simulink model "model_compatible"  (Simulink 7.5)
settings: Solver=ode45  StartTime=0.0  StopTime=10.0  RelTol=1e-3
libraries: powerlib x51
settings Model: Creator=lej  LastModifiedBy=epezhman  CovModelRefEnable=off
settings DataIOCC: SaveFormat=StructureWithTime
settings OptimizationCC: ExpressionDepthLimit=128
settings DebuggingCC: UnderspecifiedInitializationDetection=Simplified  MergeDetectMultiDrivingBlocksExec=error  SolverPrmCheckMsg=none  FcnCallInpInsideContextMsg=Enable All  StateNameClashWarn=none
settings HardwareCC: ProdIntDivRoundTo=Zero  ProdEndianess=LittleEndian  ProdHWDeviceType=Specified
settings CodeAppCC: CustomSymbolStrType=$N$R$M_T
settings GRTTargetCC: TargetFunctionLibrary=C89/C90 (ANSI)  GeneratePreprocessorConditionals=Use local settings

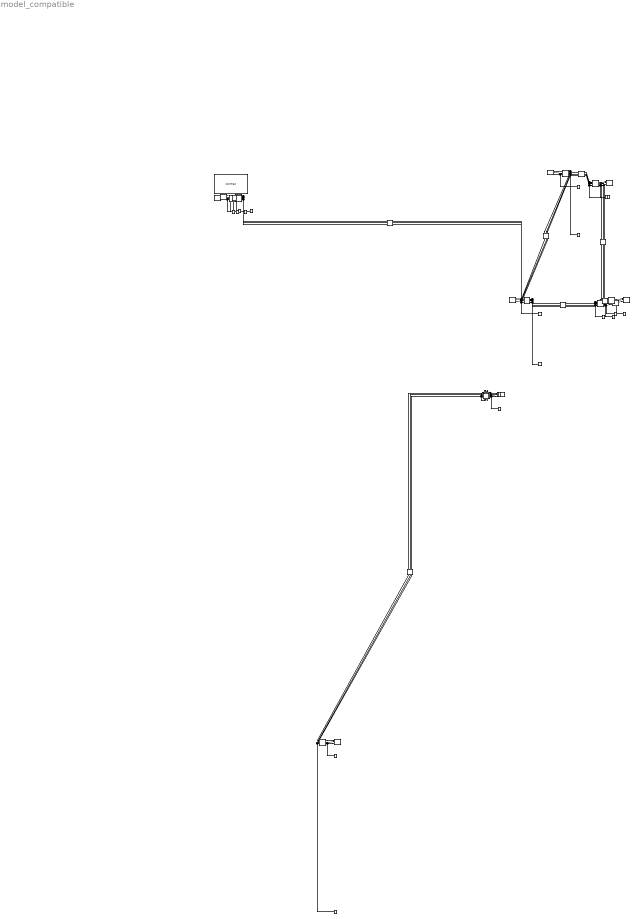
== system model_compatible ==
  note: 220000 Volts Power Line
  G_179496206_ : powerlib/Electrical Sources/Three-Phase Source  InternalConnection=Yg  VoltagePhases=off  Voltage=220000  PhaseAngle=0  Voltage_phases=[ 1 1 1]*380000  PhaseAngles_phases=[ 0 0 0]  Frequency=50  NonIdealSource=on  SpecifyImpedance=off  Resistance=0.8929  Inductance=16.58e-3  ShortCircuitLevel=100e6  BaseVoltage=220000  XRratio=7  BusType=swing  Pref=90000000  Qref=0  Prefabc=[3333.33 3333.33 3333.33]  Qrefabc=[0 0 0]  Qmin=-inf  Qmax=inf
  G_179509355_ : powerlib/Electrical Sources/Three-Phase Source  InternalConnection=Yg  VoltagePhases=off  Voltage=220000  PhaseAngle=0  Voltage_phases=[ 1 1 1]*380000  PhaseAngles_phases=[ 0 0 0]  Frequency=50  NonIdealSource=on  SpecifyImpedance=off  Resistance=0.8929  Inductance=16.58e-3  ShortCircuitLevel=100e6  BaseVoltage=220000  XRratio=7  BusType=swing  Pref=133000000  Qref=0  Prefabc=[3333.33 3333.33 3333.33]  Qrefabc=[0 0 0]  Qmin=-inf  Qmax=inf
  L_{179488572,179490334,179490336,179496196..179496198,179496204,179509359,179509364} (9 alike) : powerlib/Elements/Three-Phase Series RLC Load  LConnTagsString=A|B|C  Configuration=Y (grounded)  NominalVoltage=220000  Vabc=[1e3 1e3 1e3]  Vabcp=[1e3 1e3 1e3]  NominalFrequency=50  UnbalancedPower=off  ActivePower=100000  InductivePower=100  CapacitivePower=100  Pabc=[10e3 9e3 11e3]  QLabc=[100 90 110]  QCabc=[100 90 110]  Pabcp=[10e3 9e3 11e3]  QLabcp=[100 90 110]  QCabcp=[100 90 110]  Measurements=None  LoadType=constant PQ
  T_179488572_400000;220000_Phokoje_Substation : powerlib/Elements/Three-Phase Transformer (Two Windings)  Winding1Connection=Yg  Winding2Connection=Yg  CoreType=Three single-phase transformers  SetSaturation=off  Hysteresis=off  DataFile='hysteresis'  SetInitialFlux=off  Measurements=None  UNITS=pu  NominalPower=[ 250e6 , 50 ]  Winding1=[220000,0.002,0.08]  Winding2=[220000,0.002,0.08]  Rm=2000  Lm=50  L0=0.5  Saturation=[ 0,0 ; 0.0024,1.2 ; 1.0,1.52 ]  InitialFluxes=[ 0.8 , -0.8 , 0.7 ]  MoreParameters=off  BreakLoop=off  DataType=off  TransfoNumber=1
  T_179490334_220000_Tati_Substation : powerlib/Elements/Three-Phase Transformer (Two Windings)  Winding1Connection=Yg  Winding2Connection=Yg  CoreType=Three single-phase transformers  SetSaturation=off  Hysteresis=off  DataFile='hysteresis'  SetInitialFlux=off  Measurements=None  UNITS=pu  NominalPower=[ 250e6 , 50 ]  Winding1=[220000,0.002,0.08]  Winding2=[220000,0.002,0.08]  Rm=2000  Lm=50  L0=0.5  Saturation=[ 0,0 ; 0.0024,1.2 ; 1.0,1.52 ]  InitialFluxes=[ 0.8 , -0.8 , 0.7 ]  MoreParameters=off  BreakLoop=off  DataType=off  TransfoNumber=1
  T_179490336_220000_Francistown_Substation : powerlib/Elements/Three-Phase Transformer (Two Windings)  Winding1Connection=Yg  Winding2Connection=Yg  CoreType=Three single-phase transformers  SetSaturation=off  Hysteresis=off  DataFile='hysteresis'  SetInitialFlux=off  Measurements=None  UNITS=pu  NominalPower=[ 250e6 , 50 ]  Winding1=[220000,0.002,0.08]  Winding2=[220000,0.002,0.08]  Rm=2000  Lm=50  L0=0.5  Saturation=[ 0,0 ; 0.0024,1.2 ; 1.0,1.52 ]  InitialFluxes=[ 0.8 , -0.8 , 0.7 ]  MoreParameters=off  BreakLoop=off  DataType=off  TransfoNumber=1
  T_179496196_220000_Selebi_Pikwe_Substation : powerlib/Elements/Three-Phase Transformer (Two Windings)  Winding1Connection=Yg  Winding2Connection=Yg  CoreType=Three single-phase transformers  SetSaturation=off  Hysteresis=off  DataFile='hysteresis'  SetInitialFlux=off  Measurements=None  UNITS=pu  NominalPower=[ 250e6 , 50 ]  Winding1=[220000,0.002,0.08]  Winding2=[220000,0.002,0.08]  Rm=2000  Lm=50  L0=0.5  Saturation=[ 0,0 ; 0.0024,1.2 ; 1.0,1.52 ]  InitialFluxes=[ 0.8 , -0.8 , 0.7 ]  MoreParameters=off  BreakLoop=off  DataType=off  TransfoNumber=1
  T_179496197_220000_Orapa_Substation : powerlib/Elements/Three-Phase Transformer (Two Windings)  Winding1Connection=Yg  Winding2Connection=Yg  CoreType=Three single-phase transformers  SetSaturation=off  Hysteresis=off  DataFile='hysteresis'  SetInitialFlux=off  Measurements=None  UNITS=pu  NominalPower=[ 250e6 , 50 ]  Winding1=[220000,0.002,0.08]  Winding2=[220000,0.002,0.08]  Rm=2000  Lm=50  L0=0.5  Saturation=[ 0,0 ; 0.0024,1.2 ; 1.0,1.52 ]  InitialFluxes=[ 0.8 , -0.8 , 0.7 ]  MoreParameters=off  BreakLoop=off  DataType=off  TransfoNumber=1
  T_179496198_220000_Serule_Substation : powerlib/Elements/Three-Phase Transformer (Two Windings)  Winding1Connection=Yg  Winding2Connection=Yg  CoreType=Three single-phase transformers  SetSaturation=off  Hysteresis=off  DataFile='hysteresis'  SetInitialFlux=off  Measurements=None  UNITS=pu  NominalPower=[ 250e6 , 50 ]  Winding1=[220000,0.002,0.08]  Winding2=[220000,0.002,0.08]  Rm=2000  Lm=50  L0=0.5  Saturation=[ 0,0 ; 0.0024,1.2 ; 1.0,1.52 ]  InitialFluxes=[ 0.8 , -0.8 , 0.7 ]  MoreParameters=off  BreakLoop=off  DataType=off  TransfoNumber=1
  T_179496204_220000_Orapa_Substation : powerlib/Elements/Three-Phase Transformer (Two Windings)  Winding1Connection=Yg  Winding2Connection=Yg  CoreType=Three single-phase transformers  SetSaturation=off  Hysteresis=off  DataFile='hysteresis'  SetInitialFlux=off  Measurements=None  UNITS=pu  NominalPower=[ 250e6 , 50 ]  Winding1=[220000,0.002,0.08]  Winding2=[220000,0.002,0.08]  Rm=2000  Lm=50  L0=0.5  Saturation=[ 0,0 ; 0.0024,1.2 ; 1.0,1.52 ]  InitialFluxes=[ 0.8 , -0.8 , 0.7 ]  MoreParameters=off  BreakLoop=off  DataType=off  TransfoNumber=1
  T_179509359__ : powerlib/Elements/Three-Phase Transformer (Two Windings)  Winding1Connection=Yg  Winding2Connection=Yg  CoreType=Three single-phase transformers  SetSaturation=off  Hysteresis=off  DataFile='hysteresis'  SetInitialFlux=off  Measurements=None  UNITS=pu  NominalPower=[ 250e6 , 50 ]  Winding1=[220000,0.002,0.08]  Winding2=[220000,0.002,0.08]  Rm=2000  Lm=50  L0=0.5  Saturation=[ 0,0 ; 0.0024,1.2 ; 1.0,1.52 ]  InitialFluxes=[ 0.8 , -0.8 , 0.7 ]  MoreParameters=off  BreakLoop=off  DataType=off  TransfoNumber=1
  T_179509364_220000_Gaborone_Substation : powerlib/Elements/Three-Phase Transformer (Two Windings)  Winding1Connection=Yg  Winding2Connection=Yg  CoreType=Three single-phase transformers  SetSaturation=off  Hysteresis=off  DataFile='hysteresis'  SetInitialFlux=off  Measurements=None  UNITS=pu  NominalPower=[ 250e6 , 50 ]  Winding1=[220000,0.002,0.08]  Winding2=[220000,0.002,0.08]  Rm=2000  Lm=50  L0=0.5  Saturation=[ 0,0 ; 0.0024,1.2 ; 1.0,1.52 ]  InitialFluxes=[ 0.8 , -0.8 , 0.7 ]  MoreParameters=off  BreakLoop=off  DataType=off  TransfoNumber=1
  _CN_179488572_220000_CN_179490334_220000 : powerlib/Elements/Distributed Parameters Line  Phases=3  Frequency=50  Resistance=[0.01273 0.3864]  Inductance="[0.9337e-3  4.1264e-3]"  Capacitance=[12.74e-9 7.751e-9]  Length=84.299  x1=[8.73114913702011e-11 380000 380000;314.159265358979 314.159265358979 314.159265358979;-0.177670123217348 0.415246442777429 -1.15554988401747]  x2=[1.26090477118469e-09 381852.398472139 381852.398472139;314.159265358979 314.159265358979 314.159265358979;-1.41941675517191 0.415007521738739 -1.15578880505616]  x3=[1.07663708898761e-11 1405.24743813465 1405.24743813466;314.159265358979 314.159265358979 314.159265358979;-2.70558821102223 0.316110507002444 -1.25468581979246]  x4=[8.62234243168895e-12 1405.96374414071 1405.9637441407;314.159265358979 314.159265358979 314.159265358979;0.245769282942371 0.405640215255436 -1.16515611153945]  x5=0.000565541566995742  V1=ones(3,3)  V2=ones(3,3)  I1=ones(3,3)  I2=ones(3,3)  nHarmo=1  Measurements=None
  _CN_179490336_220000_CN_179490334_220000 : powerlib/Elements/Distributed Parameters Line  Phases=3  Frequency=50  Resistance=[0.01273 0.3864]  Inductance="[0.9337e-3  4.1264e-3]"  Capacitance=[12.74e-9 7.751e-9]  Length=27.304  x1=[8.73114913702011e-11 380000 380000;314.159265358979 314.159265358979 314.159265358979;-0.177670123217348 0.415246442777429 -1.15554988401747]  x2=[1.26090477118469e-09 381852.398472139 381852.398472139;314.159265358979 314.159265358979 314.159265358979;-1.41941675517191 0.415007521738739 -1.15578880505616]  x3=[1.07663708898761e-11 1405.24743813465 1405.24743813466;314.159265358979 314.159265358979 314.159265358979;-2.70558821102223 0.316110507002444 -1.25468581979246]  x4=[8.62234243168895e-12 1405.96374414071 1405.9637441407;314.159265358979 314.159265358979 314.159265358979;0.245769282942371 0.405640215255436 -1.16515611153945]  x5=0.000565541566995742  V1=ones(3,3)  V2=ones(3,3)  I1=ones(3,3)  I2=ones(3,3)  nHarmo=1  Measurements=None
  _CN_179490336_220000_CN_179496198_220000 : powerlib/Elements/Distributed Parameters Line  Phases=3  Frequency=50  Resistance=[0.01273 0.3864]  Inductance="[0.9337e-3  4.1264e-3]"  Capacitance=[12.74e-9 7.751e-9]  Length=92.6463  x1=[8.73114913702011e-11 380000 380000;314.159265358979 314.159265358979 314.159265358979;-0.177670123217348 0.415246442777429 -1.15554988401747]  x2=[1.26090477118469e-09 381852.398472139 381852.398472139;314.159265358979 314.159265358979 314.159265358979;-1.41941675517191 0.415007521738739 -1.15578880505616]  x3=[1.07663708898761e-11 1405.24743813465 1405.24743813466;314.159265358979 314.159265358979 314.159265358979;-2.70558821102223 0.316110507002444 -1.25468581979246]  x4=[8.62234243168895e-12 1405.96374414071 1405.9637441407;314.159265358979 314.159265358979 314.159265358979;0.245769282942371 0.405640215255436 -1.16515611153945]  x5=0.000565541566995742  V1=ones(3,3)  V2=ones(3,3)  I1=ones(3,3)  I2=ones(3,3)  nHarmo=1  Measurements=None
  _CN_179496196_220000_CN_179488572_220000 : powerlib/Elements/Distributed Parameters Line  Phases=3  Frequency=50  Resistance=[0.01273 0.3864]  Inductance="[0.9337e-3  4.1264e-3]"  Capacitance=[12.74e-9 7.751e-9]  Length=7.9024  x1=[8.73114913702011e-11 380000 380000;314.159265358979 314.159265358979 314.159265358979;-0.177670123217348 0.415246442777429 -1.15554988401747]  x2=[1.26090477118469e-09 381852.398472139 381852.398472139;314.159265358979 314.159265358979 314.159265358979;-1.41941675517191 0.415007521738739 -1.15578880505616]  x3=[1.07663708898761e-11 1405.24743813465 1405.24743813466;314.159265358979 314.159265358979 314.159265358979;-2.70558821102223 0.316110507002444 -1.25468581979246]  x4=[8.62234243168895e-12 1405.96374414071 1405.9637441407;314.159265358979 314.159265358979 314.159265358979;0.245769282942371 0.405640215255436 -1.16515611153945]  x5=0.000565541566995742  V1=ones(3,3)  V2=ones(3,3)  I1=ones(3,3)  I2=ones(3,3)  nHarmo=1  Measurements=None
  _CN_179496197_220000_CN_179496204_220000 : powerlib/Elements/Distributed Parameters Line  Phases=3  Frequency=50  Resistance=[0.01273 0.3864]  Inductance="[0.9337e-3  4.1264e-3]"  Capacitance=[12.74e-9 7.751e-9]  Length=4.007  x1=[8.73114913702011e-11 380000 380000;314.159265358979 314.159265358979 314.159265358979;-0.177670123217348 0.415246442777429 -1.15554988401747]  x2=[1.26090477118469e-09 381852.398472139 381852.398472139;314.159265358979 314.159265358979 314.159265358979;-1.41941675517191 0.415007521738739 -1.15578880505616]  x3=[1.07663708898761e-11 1405.24743813465 1405.24743813466;314.159265358979 314.159265358979 314.159265358979;-2.70558821102223 0.316110507002444 -1.25468581979246]  x4=[8.62234243168895e-12 1405.96374414071 1405.9637441407;314.159265358979 314.159265358979 314.159265358979;0.245769282942371 0.405640215255436 -1.16515611153945]  x5=0.000565541566995742  V1=ones(3,3)  V2=ones(3,3)  I1=ones(3,3)  I2=ones(3,3)  nHarmo=1  Measurements=None
  _CN_179496198_220000_CN_179488572_220000 : powerlib/Elements/Distributed Parameters Line  Phases=3  Frequency=50  Resistance=[0.01273 0.3864]  Inductance="[0.9337e-3  4.1264e-3]"  Capacitance=[12.74e-9 7.751e-9]  Length=51.2709  x1=[8.73114913702011e-11 380000 380000;314.159265358979 314.159265358979 314.159265358979;-0.177670123217348 0.415246442777429 -1.15554988401747]  x2=[1.26090477118469e-09 381852.398472139 381852.398472139;314.159265358979 314.159265358979 314.159265358979;-1.41941675517191 0.415007521738739 -1.15578880505616]  x3=[1.07663708898761e-11 1405.24743813465 1405.24743813466;314.159265358979 314.159265358979 314.159265358979;-2.70558821102223 0.316110507002444 -1.25468581979246]  x4=[8.62234243168895e-12 1405.96374414071 1405.9637441407;314.159265358979 314.159265358979 314.159265358979;0.245769282942371 0.405640215255436 -1.16515611153945]  x5=0.000565541566995742  V1=ones(3,3)  V2=ones(3,3)  I1=ones(3,3)  I2=ones(3,3)  nHarmo=1  Measurements=None
  _CN_179496198_220000_CN_179496204_220000 : powerlib/Elements/Distributed Parameters Line  Phases=3  Frequency=50  Resistance=[0.01273 0.3864]  Inductance="[0.9337e-3  4.1264e-3]"  Capacitance=[12.74e-9 7.751e-9]  Length=33.2853  x1=[8.73114913702011e-11 380000 380000;314.159265358979 314.159265358979 314.159265358979;-0.177670123217348 0.415246442777429 -1.15554988401747]  x2=[1.26090477118469e-09 381852.398472139 381852.398472139;314.159265358979 314.159265358979 314.159265358979;-1.41941675517191 0.415007521738739 -1.15578880505616]  x3=[1.07663708898761e-11 1405.24743813465 1405.24743813466;314.159265358979 314.159265358979 314.159265358979;-2.70558821102223 0.316110507002444 -1.25468581979246]  x4=[8.62234243168895e-12 1405.96374414071 1405.9637441407;314.159265358979 314.159265358979 314.159265358979;0.245769282942371 0.405640215255436 -1.16515611153945]  x5=0.000565541566995742  V1=ones(3,3)  V2=ones(3,3)  I1=ones(3,3)  I2=ones(3,3)  nHarmo=1  Measurements=None
  _CN_179496204_220000_CN_179496206_220000 : powerlib/Elements/Distributed Parameters Line  Phases=3  Frequency=50  Resistance=[0.01273 0.3864]  Inductance="[0.9337e-3  4.1264e-3]"  Capacitance=[12.74e-9 7.751e-9]  Length=0.29284  x1=[8.73114913702011e-11 380000 380000;314.159265358979 314.159265358979 314.159265358979;-0.177670123217348 0.415246442777429 -1.15554988401747]  x2=[1.26090477118469e-09 381852.398472139 381852.398472139;314.159265358979 314.159265358979 314.159265358979;-1.41941675517191 0.415007521738739 -1.15578880505616]  x3=[1.07663708898761e-11 1405.24743813465 1405.24743813466;314.159265358979 314.159265358979 314.159265358979;-2.70558821102223 0.316110507002444 -1.25468581979246]  x4=[8.62234243168895e-12 1405.96374414071 1405.9637441407;314.159265358979 314.159265358979 314.159265358979;0.245769282942371 0.405640215255436 -1.16515611153945]  x5=0.000565541566995742  V1=ones(3,3)  V2=ones(3,3)  I1=ones(3,3)  I2=ones(3,3)  nHarmo=1  Measurements=None
  _CN_179509359_220000_CN_179509355_220000 : powerlib/Elements/Distributed Parameters Line  Phases=3  Frequency=50  Resistance=[0.01273 0.3864]  Inductance="[0.9337e-3  4.1264e-3]"  Capacitance=[12.74e-9 7.751e-9]  Length=0.14091  x1=[8.73114913702011e-11 380000 380000;314.159265358979 314.159265358979 314.159265358979;-0.177670123217348 0.415246442777429 -1.15554988401747]  x2=[1.26090477118469e-09 381852.398472139 381852.398472139;314.159265358979 314.159265358979 314.159265358979;-1.41941675517191 0.415007521738739 -1.15578880505616]  x3=[1.07663708898761e-11 1405.24743813465 1405.24743813466;314.159265358979 314.159265358979 314.159265358979;-2.70558821102223 0.316110507002444 -1.25468581979246]  x4=[8.62234243168895e-12 1405.96374414071 1405.9637441407;314.159265358979 314.159265358979 314.159265358979;0.245769282942371 0.405640215255436 -1.16515611153945]  x5=0.000565541566995742  V1=ones(3,3)  V2=ones(3,3)  I1=ones(3,3)  I2=ones(3,3)  nHarmo=1  Measurements=None
  _CN_179509364_220000_CN_179509355_220000 : powerlib/Elements/Distributed Parameters Line  Phases=3  Frequency=50  Resistance=[0.01273 0.3864]  Inductance="[0.9337e-3  4.1264e-3]"  Capacitance=[12.74e-9 7.751e-9]  Length=172.4004  x1=[8.73114913702011e-11 380000 380000;314.159265358979 314.159265358979 314.159265358979;-0.177670123217348 0.415246442777429 -1.15554988401747]  x2=[1.26090477118469e-09 381852.398472139 381852.398472139;314.159265358979 314.159265358979 314.159265358979;-1.41941675517191 0.415007521738739 -1.15578880505616]  x3=[1.07663708898761e-11 1405.24743813465 1405.24743813466;314.159265358979 314.159265358979 314.159265358979;-2.70558821102223 0.316110507002444 -1.25468581979246]  x4=[8.62234243168895e-12 1405.96374414071 1405.9637441407;314.159265358979 314.159265358979 314.159265358979;0.245769282942371 0.405640215255436 -1.16515611153945]  x5=0.000565541566995742  V1=ones(3,3)  V2=ones(3,3)  I1=ones(3,3)  I2=ones(3,3)  nHarmo=1  Measurements=None
  bus1 : powerlib/Measurements/Load Flow Bus  LConnTagsString=a  Phases=single  Connectors=on one side  ID=bus1  Vbase=220000  Vref=1  Vangle=0  VLF=1  VLFb=1  VLFc=1  angleLF=0  angleLFb=0  angleLFc=0
      settings: AttributesFormatString=|
      | %<ID>
      | %<Vbase>V
      | %<VLF>pu
      | %<angleLF>deg.
      | %<Name>
  bus10 : powerlib/Measurements/Load Flow Bus  LConnTagsString=a  Phases=single  Connectors=on one side  ID=bus10  Vbase=220000  Vref=1  Vangle=0  VLF=1  VLFb=1  VLFc=1  angleLF=0  angleLFb=0  angleLFc=0
      settings: AttributesFormatString=|
      | %<ID>
      | %<Vbase>V
      | %<VLF>pu
      | %<angleLF>deg.
      | %<Name>
  bus11 : powerlib/Measurements/Load Flow Bus  LConnTagsString=a  Phases=single  Connectors=on one side  ID=bus11  Vbase=220000  Vref=1  Vangle=0  VLF=1  VLFb=1  VLFc=1  angleLF=0  angleLFb=0  angleLFc=0
      settings: AttributesFormatString=|
      | %<ID>
      | %<Vbase>V
      | %<VLF>pu
      | %<angleLF>deg.
      | %<Name>
  bus12 : powerlib/Measurements/Load Flow Bus  LConnTagsString=a  Phases=single  Connectors=on one side  ID=bus12  Vbase=220000  Vref=1  Vangle=0  VLF=1  VLFb=1  VLFc=1  angleLF=0  angleLFb=0  angleLFc=0
      settings: AttributesFormatString=|
      | %<ID>
      | %<Vbase>V
      | %<VLF>pu
      | %<angleLF>deg.
      | %<Name>
  bus13 : powerlib/Measurements/Load Flow Bus  LConnTagsString=a  Phases=single  Connectors=on one side  ID=bus13  Vbase=220000  Vref=1  Vangle=0  VLF=1  VLFb=1  VLFc=1  angleLF=0  angleLFb=0  angleLFc=0
      settings: AttributesFormatString=|
      | %<ID>
      | %<Vbase>V
      | %<VLF>pu
      | %<angleLF>deg.
      | %<Name>
  bus14 : powerlib/Measurements/Load Flow Bus  LConnTagsString=a  Phases=single  Connectors=on one side  ID=bus14  Vbase=220000  Vref=1  Vangle=0  VLF=1  VLFb=1  VLFc=1  angleLF=0  angleLFb=0  angleLFc=0
      settings: AttributesFormatString=|
      | %<ID>
      | %<Vbase>V
      | %<VLF>pu
      | %<angleLF>deg.
      | %<Name>
  bus15 : powerlib/Measurements/Load Flow Bus  LConnTagsString=a  Phases=single  Connectors=on one side  ID=bus15  Vbase=220000  Vref=1  Vangle=0  VLF=1  VLFb=1  VLFc=1  angleLF=0  angleLFb=0  angleLFc=0
      settings: AttributesFormatString=|
      | %<ID>
      | %<Vbase>V
      | %<VLF>pu
      | %<angleLF>deg.
      | %<Name>
  bus16 : powerlib/Measurements/Load Flow Bus  LConnTagsString=a  Phases=single  Connectors=on one side  ID=bus16  Vbase=220000  Vref=1  Vangle=0  VLF=1  VLFb=1  VLFc=1  angleLF=0  angleLFb=0  angleLFc=0
      settings: AttributesFormatString=|
      | %<ID>
      | %<Vbase>V
      | %<VLF>pu
      | %<angleLF>deg.
      | %<Name>
  bus17 : powerlib/Measurements/Load Flow Bus  LConnTagsString=a  Phases=single  Connectors=on one side  ID=bus17  Vbase=220000  Vref=1  Vangle=0  VLF=1  VLFb=1  VLFc=1  angleLF=0  angleLFb=0  angleLFc=0
      settings: AttributesFormatString=|
      | %<ID>
      | %<Vbase>V
      | %<VLF>pu
      | %<angleLF>deg.
      | %<Name>
  bus18 : powerlib/Measurements/Load Flow Bus  LConnTagsString=a  Phases=single  Connectors=on one side  ID=bus18  Vbase=220000  Vref=1  Vangle=0  VLF=1  VLFb=1  VLFc=1  angleLF=0  angleLFb=0  angleLFc=0
      settings: AttributesFormatString=|
      | %<ID>
      | %<Vbase>V
      | %<VLF>pu
      | %<angleLF>deg.
      | %<Name>
  bus19 : powerlib/Measurements/Load Flow Bus  LConnTagsString=a  Phases=single  Connectors=on one side  ID=bus19  Vbase=220000  Vref=1  Vangle=0  VLF=1  VLFb=1  VLFc=1  angleLF=0  angleLFb=0  angleLFc=0
      settings: AttributesFormatString=|
      | %<ID>
      | %<Vbase>V
      | %<VLF>pu
      | %<angleLF>deg.
      | %<Name>
  bus2 : powerlib/Measurements/Load Flow Bus  LConnTagsString=a  Phases=single  Connectors=on one side  ID=bus2  Vbase=220000  Vref=1  Vangle=0  VLF=1  VLFb=1  VLFc=1  angleLF=0  angleLFb=0  angleLFc=0
      settings: AttributesFormatString=|
      | %<ID>
      | %<Vbase>V
      | %<VLF>pu
      | %<angleLF>deg.
      | %<Name>
  bus20 : powerlib/Measurements/Load Flow Bus  LConnTagsString=a  Phases=single  Connectors=on one side  ID=bus20  Vbase=220000  Vref=1  Vangle=0  VLF=1  VLFb=1  VLFc=1  angleLF=0  angleLFb=0  angleLFc=0
      settings: AttributesFormatString=|
      | %<ID>
      | %<Vbase>V
      | %<VLF>pu
      | %<angleLF>deg.
      | %<Name>
  bus3 : powerlib/Measurements/Load Flow Bus  LConnTagsString=a  Phases=single  Connectors=on one side  ID=bus3  Vbase=220000  Vref=1  Vangle=0  VLF=1  VLFb=1  VLFc=1  angleLF=0  angleLFb=0  angleLFc=0
      settings: AttributesFormatString=|
      | %<ID>
      | %<Vbase>V
      | %<VLF>pu
      | %<angleLF>deg.
      | %<Name>
  bus4 : powerlib/Measurements/Load Flow Bus  LConnTagsString=a  Phases=single  Connectors=on one side  ID=bus4  Vbase=220000  Vref=1  Vangle=0  VLF=1  VLFb=1  VLFc=1  angleLF=0  angleLFb=0  angleLFc=0
      settings: AttributesFormatString=|
      | %<ID>
      | %<Vbase>V
      | %<VLF>pu
      | %<angleLF>deg.
      | %<Name>
  bus5 : powerlib/Measurements/Load Flow Bus  LConnTagsString=a  Phases=single  Connectors=on one side  ID=bus5  Vbase=220000  Vref=1  Vangle=0  VLF=1  VLFb=1  VLFc=1  angleLF=0  angleLFb=0  angleLFc=0
      settings: AttributesFormatString=|
      | %<ID>
      | %<Vbase>V
      | %<VLF>pu
      | %<angleLF>deg.
      | %<Name>
  bus6 : powerlib/Measurements/Load Flow Bus  LConnTagsString=a  Phases=single  Connectors=on one side  ID=bus6  Vbase=220000  Vref=1  Vangle=0  VLF=1  VLFb=1  VLFc=1  angleLF=0  angleLFb=0  angleLFc=0
      settings: AttributesFormatString=|
      | %<ID>
      | %<Vbase>V
      | %<VLF>pu
      | %<angleLF>deg.
      | %<Name>
  bus7 : powerlib/Measurements/Load Flow Bus  LConnTagsString=a  Phases=single  Connectors=on one side  ID=bus7  Vbase=220000  Vref=1  Vangle=0  VLF=1  VLFb=1  VLFc=1  angleLF=0  angleLFb=0  angleLFc=0
      settings: AttributesFormatString=|
      | %<ID>
      | %<Vbase>V
      | %<VLF>pu
      | %<angleLF>deg.
      | %<Name>
  bus8 : powerlib/Measurements/Load Flow Bus  LConnTagsString=a  Phases=single  Connectors=on one side  ID=bus8  Vbase=220000  Vref=1  Vangle=0  VLF=1  VLFb=1  VLFc=1  angleLF=0  angleLFb=0  angleLFc=0
      settings: AttributesFormatString=|
      | %<ID>
      | %<Vbase>V
      | %<VLF>pu
      | %<angleLF>deg.
      | %<Name>
  bus9 : powerlib/Measurements/Load Flow Bus  LConnTagsString=a  Phases=single  Connectors=on one side  ID=bus9  Vbase=220000  Vref=1  Vangle=0  VLF=1  VLFb=1  VLFc=1  angleLF=0  angleLFb=0  angleLFc=0
      settings: AttributesFormatString=|
      | %<ID>
      | %<Vbase>V
      | %<VLF>pu
      | %<angleLF>deg.
      | %<Name>
  powergui : powerlib/powergui  Priority=1  SimulationMode=Phasor  SolverType=Tustin/Backward Euler (TBE)  SampleTime=50e-6  frequency=50  SPID=off  DisableSnubberDevices=off  DisableRonSwitches=off  DisableVfSwitches=off  SwTol=0  DisplayEquations=off  Interpol=off  ExternalGateDelay=off  methode=off  Ts=10  FunctionMessages=off  echomessages=off  HookPort=off  EnableUseOfTLC=off  x0status=blocks  frequencyindice=50  Pbase=3000e6  ErrMax=0.0001  Iterations=50  UnitsV=V  UnitsW=W  buscounter=0  RestoreLinks=warning  ResistiveCurrentMeasurement=off  Frange=[0:2:500]  Ylog=off  Xlog=on  ShowGrid=off  save=off  variable=ZData  structure=0  ZoomFFT=off  StartTime=0.0  cycles=1  DisplayStyle=1  fundamental=60  FreqAxis=off  MaxFrequency=1000  frequencyindicesteady=1  RmsSteady=1  display=off
  connections:
  _CN_179490336_220000_CN_179496198_220000/LConn1 -- T_179490336_220000_Francistown_Substation/LConn1 -- _CN_179490336_220000_CN_179490334_220000/LConn1
  _CN_179490336_220000_CN_179496198_220000/LConn2 -- T_179490336_220000_Francistown_Substation/LConn2 -- _CN_179490336_220000_CN_179490334_220000/LConn2
  _CN_179490336_220000_CN_179496198_220000/LConn3 -- T_179490336_220000_Francistown_Substation/LConn3 -- _CN_179490336_220000_CN_179490334_220000/LConn3 -- bus1/LConn1
  _CN_179490336_220000_CN_179496198_220000/RConn1 -- T_179496198_220000_Serule_Substation/LConn1 -- _CN_179496198_220000_CN_179488572_220000/LConn1 -- _CN_179496198_220000_CN_179496204_220000/LConn1
  _CN_179490336_220000_CN_179496198_220000/RConn2 -- T_179496198_220000_Serule_Substation/LConn2 -- _CN_179496198_220000_CN_179488572_220000/LConn2 -- _CN_179496198_220000_CN_179496204_220000/LConn2
  _CN_179490336_220000_CN_179496198_220000/RConn3 -- T_179496198_220000_Serule_Substation/LConn3 -- _CN_179496198_220000_CN_179488572_220000/LConn3 -- bus2/LConn1 -- _CN_179496198_220000_CN_179496204_220000/LConn3
  _CN_179490336_220000_CN_179490334_220000/RConn1 -- T_179490334_220000_Tati_Substation/LConn1 -- _CN_179488572_220000_CN_179490334_220000/LConn1
  _CN_179490336_220000_CN_179490334_220000/RConn2 -- T_179490334_220000_Tati_Substation/LConn2 -- _CN_179488572_220000_CN_179490334_220000/LConn2
  _CN_179490336_220000_CN_179490334_220000/RConn3 -- T_179490334_220000_Tati_Substation/LConn3 -- _CN_179488572_220000_CN_179490334_220000/LConn3 -- bus3/LConn1
  T_179496196_220000_Selebi_Pikwe_Substation/LConn1 -- _CN_179496196_220000_CN_179488572_220000/LConn1
  T_179496196_220000_Selebi_Pikwe_Substation/LConn2 -- _CN_179496196_220000_CN_179488572_220000/LConn2
  _CN_179496196_220000_CN_179488572_220000/LConn3 -- T_179496196_220000_Selebi_Pikwe_Substation/LConn3 -- bus4/LConn1
  _CN_179496196_220000_CN_179488572_220000/RConn1 -- T_179488572_400000;220000_Phokoje_Substation/LConn1 -- _CN_179496198_220000_CN_179488572_220000/RConn1 -- _CN_179488572_220000_CN_179490334_220000/RConn1
  _CN_179496196_220000_CN_179488572_220000/RConn2 -- T_179488572_400000;220000_Phokoje_Substation/LConn2 -- _CN_179496198_220000_CN_179488572_220000/RConn2 -- _CN_179488572_220000_CN_179490334_220000/RConn2
  _CN_179496196_220000_CN_179488572_220000/RConn3 -- T_179488572_400000;220000_Phokoje_Substation/LConn3 -- _CN_179496198_220000_CN_179488572_220000/RConn3 -- _CN_179488572_220000_CN_179490334_220000/RConn3 -- bus5/LConn1
  T_179496197_220000_Orapa_Substation/LConn1 -- _CN_179496197_220000_CN_179496204_220000/LConn1
  T_179496197_220000_Orapa_Substation/LConn2 -- _CN_179496197_220000_CN_179496204_220000/LConn2
  _CN_179496197_220000_CN_179496204_220000/LConn3 -- T_179496197_220000_Orapa_Substation/LConn3 -- bus6/LConn1
  _CN_179496197_220000_CN_179496204_220000/RConn1 -- T_179496204_220000_Orapa_Substation/LConn1 -- _CN_179496198_220000_CN_179496204_220000/RConn1 -- _CN_179496204_220000_CN_179496206_220000/LConn1
  _CN_179496197_220000_CN_179496204_220000/RConn2 -- T_179496204_220000_Orapa_Substation/LConn2 -- _CN_179496198_220000_CN_179496204_220000/RConn2 -- _CN_179496204_220000_CN_179496206_220000/LConn2
  _CN_179496197_220000_CN_179496204_220000/RConn3 -- T_179496204_220000_Orapa_Substation/LConn3 -- _CN_179496198_220000_CN_179496204_220000/RConn3 -- _CN_179496204_220000_CN_179496206_220000/LConn3 -- bus7/LConn1
  G_179496206_/RConn1 -- _CN_179496204_220000_CN_179496206_220000/RConn1
  G_179496206_/RConn2 -- _CN_179496204_220000_CN_179496206_220000/RConn2
  _CN_179496204_220000_CN_179496206_220000/RConn3 -- G_179496206_/RConn3 -- bus8/LConn1
  T_179509359__/LConn1 -- _CN_179509359_220000_CN_179509355_220000/LConn1
  T_179509359__/LConn2 -- _CN_179509359_220000_CN_179509355_220000/LConn2
  _CN_179509359_220000_CN_179509355_220000/LConn3 -- T_179509359__/LConn3 -- bus9/LConn1
  _CN_179509359_220000_CN_179509355_220000/RConn1 -- G_179509355_/RConn1 -- _CN_179509364_220000_CN_179509355_220000/LConn1
  _CN_179509359_220000_CN_179509355_220000/RConn2 -- G_179509355_/RConn2 -- _CN_179509364_220000_CN_179509355_220000/LConn2
  _CN_179509359_220000_CN_179509355_220000/RConn3 -- G_179509355_/RConn3 -- _CN_179509364_220000_CN_179509355_220000/LConn3 -- bus10/LConn1
  T_179509364_220000_Gaborone_Substation/LConn1 -- _CN_179509364_220000_CN_179509355_220000/RConn1
  T_179509364_220000_Gaborone_Substation/LConn2 -- _CN_179509364_220000_CN_179509355_220000/RConn2
  _CN_179509364_220000_CN_179509355_220000/RConn3 -- T_179509364_220000_Gaborone_Substation/LConn3 -- bus11/LConn1
  T_179490336_220000_Francistown_Substation/RConn1 -- L_179490336/LConn1
  T_179490336_220000_Francistown_Substation/RConn2 -- L_179490336/LConn2
  L_179490336/LConn3 -- T_179490336_220000_Francistown_Substation/RConn3 -- bus12/LConn1
  T_179496198_220000_Serule_Substation/RConn1 -- L_179496198/LConn1
  T_179496198_220000_Serule_Substation/RConn2 -- L_179496198/LConn2
  L_179496198/LConn3 -- T_179496198_220000_Serule_Substation/RConn3 -- bus13/LConn1
  T_179490334_220000_Tati_Substation/RConn1 -- L_179490334/LConn1
  T_179490334_220000_Tati_Substation/RConn2 -- L_179490334/LConn2
  L_179490334/LConn3 -- T_179490334_220000_Tati_Substation/RConn3 -- bus14/LConn1
  T_179496196_220000_Selebi_Pikwe_Substation/RConn1 -- L_179496196/LConn1
  T_179496196_220000_Selebi_Pikwe_Substation/RConn2 -- L_179496196/LConn2
  L_179496196/LConn3 -- T_179496196_220000_Selebi_Pikwe_Substation/RConn3 -- bus15/LConn1
  T_179488572_400000;220000_Phokoje_Substation/RConn1 -- L_179488572/LConn1
  T_179488572_400000;220000_Phokoje_Substation/RConn2 -- L_179488572/LConn2
  L_179488572/LConn3 -- T_179488572_400000;220000_Phokoje_Substation/RConn3 -- bus16/LConn1
  T_179496197_220000_Orapa_Substation/RConn1 -- L_179496197/LConn1
  T_179496197_220000_Orapa_Substation/RConn2 -- L_179496197/LConn2
  L_179496197/LConn3 -- T_179496197_220000_Orapa_Substation/RConn3 -- bus17/LConn1
  T_179496204_220000_Orapa_Substation/RConn1 -- L_179496204/LConn1
  T_179496204_220000_Orapa_Substation/RConn2 -- L_179496204/LConn2
  L_179496204/LConn3 -- T_179496204_220000_Orapa_Substation/RConn3 -- bus18/LConn1
  T_179509359__/RConn1 -- L_179509359/LConn1
  T_179509359__/RConn2 -- L_179509359/LConn2
  L_179509359/LConn3 -- T_179509359__/RConn3 -- bus19/LConn1
  T_179509364_220000_Gaborone_Substation/RConn1 -- L_179509364/LConn1
  T_179509364_220000_Gaborone_Substation/RConn2 -- L_179509364/LConn2
  L_179509364/LConn3 -- T_179509364_220000_Gaborone_Substation/RConn3 -- bus20/LConn1
